simulink model "model_graphicSim"  (R2022a)
settings: Solver=FixedStepAuto  StartTime=0.0  StopTime=inf  RelTol=1e-3
values from neighbouring files (symbols this model uses):
  A = 9    [A_circuit_V2_25000.mat]    (also in A_circuit_V2_3167.mat; A_circuit_V3_30000.mat; A_circuit_V3_60000.mat; Configuration.m)
  d = 699840    [A_circuit_V2_25000.mat]    (also in A_circuit_V2_3167.mat; A_circuit_V3_30000.mat; A_circuit_V3_60000.mat; Configuration.m)
  egoID = 1    [A_circuit_V2_25000.mat]    (also in A_circuit_V2_3167.mat; A_circuit_V3_30000.mat; A_circuit_V3_60000.mat; Configuration.m)
  frontDistCG = 3.7    [A_circuit_V2_25000.mat]    (also in A_circuit_V2_3167.mat; A_circuit_V3_30000.mat; A_circuit_V3_60000.mat; Configuration.m)
  gridvx = [-5 -4.72222222222 -4.44444444444 -4.16666666667 -3.88888888889 -3.61111111111 -3.33333333333 -3.05555555556 -2.77777777778 -2.5 0 0.277777777778 ... (70 elements, 10x7)]    [A_circuit_V2_25000.mat]    (also in A_circuit_V2_3167.mat; A_circuit_V3_30000.mat; A_circuit_V3_60000.mat; circuit_10000_P2.mat)
  gridvy = [-70 -68.4444444444 -66.8888888889 -65.3333333333 -63.7777777778 -62.2222222222 -60.6666666667 -59.1111111111 -57.5555555556 -56 -50 -48.4444444444 ... (70 elements, 10x7)]    [A_circuit_V2_25000.mat]    (also in A_circuit_V2_3167.mat; A_circuit_V3_30000.mat; A_circuit_V3_60000.mat; circuit_10000_P2.mat)
  gridx = [-85 -84.6666666667 -84.3333333333 -84 -83.6666666667 -83.3333333333 -83 -82.6666666667 -82.3333333333 -82 -55 -54.6666666667 ... (70 elements, 10x7)]    [A_circuit_V2_25000.mat]    (also in A_circuit_V2_3167.mat; A_circuit_V3_30000.mat; A_circuit_V3_60000.mat; circuit_10000_P2.mat)
  gridy = [-70 -69.3333333333 -68.6666666667 -68 -67.3333333333 -66.6666666667 -66 -65.3333333333 -64.6666666667 -64 -50 -49.3333333333 ... (70 elements, 10x7)]    [A_circuit_V2_25000.mat]    (also in A_circuit_V2_3167.mat; A_circuit_V3_30000.mat; A_circuit_V3_60000.mat; circuit_10000_P2.mat)
  gridyaw = [-504 -489.6 -475.2 -460.8 -446.4 -432 -417.6 -403.2 -388.8 -374.4 -360 -345.6 ... (70 elements, 10x7)]    [A_circuit_V2_25000.mat]    (also in A_circuit_V2_3167.mat; A_circuit_V3_30000.mat; A_circuit_V3_60000.mat; circuit_10000_P2.mat)
  lb_angSt = -1080    [A_circuit_V2_25000.mat]    (also in A_circuit_V2_3167.mat; A_circuit_V3_30000.mat; A_circuit_V3_60000.mat; Configuration.m = -900)
  lbvx = 0    [A_circuit_V2_25000.mat]    (also in A_circuit_V2_3167.mat; A_circuit_V3_30000.mat; A_circuit_V3_60000.mat; Configuration.m = -2)
  lbvy = -50    [A_circuit_V2_25000.mat]    (also in A_circuit_V2_3167.mat; A_circuit_V3_30000.mat; A_circuit_V3_60000.mat; Configuration.m = -20)
  lbx = -55    [A_circuit_V2_25000.mat]    (also in A_circuit_V2_3167.mat; A_circuit_V3_30000.mat; A_circuit_V3_60000.mat; Configuration.m = 0)
  lby = -50    [A_circuit_V2_25000.mat]    (also in A_circuit_V2_3167.mat; A_circuit_V3_30000.mat; A_circuit_V3_60000.mat; Configuration.m = 2)
  lbyaw = -90    [Configuration.m]    (also in Configuration_circuit.m = -360; Configuration_circuit_V2.m = -360; Configuration_curve.m = -360; Configuration_curve_2.m = -360)
  leftDistCG = 0.9    [A_circuit_V2_25000.mat]    (also in A_circuit_V2_3167.mat; A_circuit_V3_30000.mat; A_circuit_V3_60000.mat; Configuration.m)
  M = 5    [A_circuit_V2_25000.mat]    (also in A_circuit_V2_3167.mat; A_circuit_V3_30000.mat; A_circuit_V3_60000.mat; Configuration.m)
  N = 10    [A_circuit_V2_25000.mat]    (also in A_circuit_V2_3167.mat; A_circuit_V3_30000.mat; A_circuit_V3_60000.mat; Configuration.m)
  passo_steerang = 45    [A_circuit_V2_25000.mat]    (also in A_circuit_V2_3167.mat; A_circuit_V3_30000.mat; A_circuit_V3_60000.mat; Configuration.m = 180)
  passo_v = 0.5    [A_circuit_V2_25000.mat]    (also in A_circuit_V2_3167.mat; A_circuit_V3_30000.mat; A_circuit_V3_60000.mat; Configuration.m)
  retroDistCG = 1    [A_circuit_V2_25000.mat]    (also in A_circuit_V2_3167.mat; A_circuit_V3_30000.mat; A_circuit_V3_60000.mat; Configuration.m)
  safetyDist = 0.5    [A_circuit_V2_25000.mat]    (also in A_circuit_V2_3167.mat; A_circuit_V3_30000.mat; A_circuit_V3_60000.mat; Configuration.m)
  Ts = 0.1    [A_circuit_V2_25000.mat]    (also in A_circuit_V2_3167.mat; A_circuit_V3_30000.mat; A_circuit_V3_60000.mat; Configuration.m)
  ub_angSt = 1080    [A_circuit_V2_25000.mat]    (also in A_circuit_V2_3167.mat; A_circuit_V3_30000.mat; A_circuit_V3_60000.mat; Configuration.m = 900)
  ubvx = 25    [A_circuit_V2_25000.mat]    (also in A_circuit_V2_3167.mat; A_circuit_V3_30000.mat; A_circuit_V3_60000.mat; Configuration.m = 2)
  ubvy = 50    [A_circuit_V2_25000.mat]    (also in A_circuit_V2_3167.mat; A_circuit_V3_30000.mat; A_circuit_V3_60000.mat; Configuration.m = 20)
  ubx = 95    [A_circuit_V2_25000.mat]    (also in A_circuit_V2_3167.mat; A_circuit_V3_30000.mat; A_circuit_V3_60000.mat; Configuration.m = 25)
  uby = 50    [A_circuit_V2_25000.mat]    (also in A_circuit_V2_3167.mat; A_circuit_V3_30000.mat; A_circuit_V3_60000.mat; Configuration.m = 10)
  ubyaw = 90    [Configuration.m]    (also in Configuration_circuit.m = 360; Configuration_circuit_V2.m = 360; Configuration_curve.m = 360; Configuration_curve_2.m = 360)
  w = [0 0 0 0 0 0 0 0 0 0 0 0 ... (699840 elements, 699840x1)]    [A_circuit_V2_25000.mat]    (also in A_circuit_V2_3167.mat; A_circuit_V3_30000.mat; A_circuit_V3_60000.mat; circuit_10000_P2.mat)
  x_0 = 2*rand+19    [Configuration.m]    (also in Configuration_circuit.m = -30; Configuration_circuit_V2.m = 0; Configuration_curve.m = 5; Configuration_curve_2.m = 5)
  y_0 = -(3.5*rand+2)    [Configuration.m]    (also in Configuration_circuit.m = -(-20 - rand*6); Configuration_circuit_V2.m = -(-29.5 - rand*7); Configuration_curve.m = -(1-2.1*rand); Configuration_curve_2.m = -(1-2.1*rand))
undefined symbols (not defined in the file or in its folder): deg, driving, rad, s
libraries: drivingscenarioandsensors x17, simulink_extras x2, sim3dlib x1, sim3dautolib x1, aerolibconvert2 x1, vehdynlibsteering x1, autolibshared x1
(part 6 of 6)

== matlab function model_graphicSim/next_a ==
  data: s input; a1 output; gridx parameter; gridy parameter; gridvx parameter; gridvy parameter; gridyaw parameter; M parameter; N parameter; A parameter; d parameter; eps parameter; w parameter; a2 output
function [a1,a2] = eps_greedy(s, gridx, gridy, gridvx, gridvy, gridyaw, M, N, A, d, eps, w)

%s(5) = -s(5);

if rand < eps   % azione random
    a = randi(A); % da 1 a 9 se uso indice
else
    q = zeros(A, 1);
    for a = 1:A  % valuto tutte le azioni che posso prendere
        q(a) = w'*get_features(s, a, gridx, gridy, gridvx, gridvy, gridyaw, M, N, A, d); % approsimazione della funz qualità
    end        % pesi per vett features
    a = find(q == max(q), 1, 'first'); % scelgo quella con funz qualità massima
end

[b1,b2] = ind2sub([3 3],a);

% [1 2 3] vanno mappati su -1,0, con (-2)

if(b1 == 1)
    a1 = 1;
elseif(b1 == 2)
    a1 = 2;
else
    a1 = 3;
end

if(b2 == 1)
    a2 = 1;
elseif(b2 == 2)
    a2 = 2;
else
    a2 = 3;
end

end


function x = get_features(s, a, gridx, gridy, gridvx, gridvy, gridyaw, M, N, A, d)

%coder.extrinsic('assignin')

% numero celle, +1 perchè ne ho aggiunta una
%nCells = (M + 1)^4; % dimensione features per una cella
%d = A*N*nCells; % dimensione vettore pesi da aggiornare
x = zeros(d, 1);
% va modificaro sta dimension var
for ii = 1 : N
    xxx = gridx(ii, :);
    yyy = gridy(ii, :);
    vxvxvx = gridvx(ii, :);
    vyvyvy = gridvy(ii, :);
    yawyawyaw = gridyaw(ii, :);
    % capire in quale cella mi trovo, trovo indice lungo x e lungo y
    ix = find(s(1) >= xxx(1:end-1) & s(1) <= xxx(2:end), 1, 'first');
    iy = find(s(2) >= yyy(1:end-1) & s(2) <= yyy(2:end), 1, 'first');
    ivx = find(s(3) >= vxvxvx(1:end-1) & s(3) <= vxvxvx(2:end), 1, 'first');
    ivy = find(s(4) >= vyvyvy(1:end-1) & s(4) <= vyvyvy(2:end), 1, 'first');
    iyaw = find(s(5) >= yawyawyaw(1:end-1) & s(5) <= yawyawyaw(2:end), 1, 'first');

    % a_ind = sub2ind([3 3],a(1),a(2)); non serve gli passo indice poi da
    % indice a azione quando la uso in dinamica
    % dato doppia dim dell'azione devo subind anche a ???

    % debug
    %pippo = struct('ix',{ix},'iy', {iy},'ivx', {ivx},'ivy', {ivy},'ii', {ii},'a', {a},'s', {s});
    %assignin("base","pippo",pippo);
    % ind = sub2ind([M + 1, M + 1, M + 1, M + 1, N, A], ix, iy, ivx, ivy, ii, a);
    ind = sub2ind([M + 1, M + 1, M + 1, M + 1, M + 1, N, A], ix, iy, ivx, ivy, iyaw, ii, a);

    x(ind) = 1; % valore corrispondente alla cella
    % vett features ha un 1 per ogni griglia
end
end

== matlab function model_graphicSim/Reward ==
  data: sp output; next_state input; RadR input; RadF input; RadSx input; RadDx input; camL_L input; camF_L input; camR_L input; r output; isTerminal output; safetyDist parameter; leftDistCG parameter; frontDistCG parameter; retroDistCG parameter; ubx parameter; lbx parameter; uby parameter; ubyaw parameter; lbyaw parameter; lby parameter
% sensori camera hanno difficoltà con ostacoli ravvicinati -> provare radar
function [sp , r, isTerminal] = reward(next_state, RadR, RadF, RadSx, RadDx, camL_L, camF_L, camR_L, safetyDist, leftDistCG, frontDistCG, retroDistCG, ubx, lbx, uby, ubyaw, lbyaw, lby)

% isTerminal quadno crash, quando fuori da ambiente -> r = r - 1000
% isTerminal qunado raggiungo distanza limite dal bordo -> r = 0
% altrimenti r = r - 1

% CG centro asse posteriore

sp = next_state;

% controllo posizione non fuori dai limiti (next_state = [x y vx vy])
% limiti ambiente statici, definirli come parametri da workspace
% if((next_state(1) < 0) || (next_state(1) > 25) || (next_state(2) < -10) || (next_state(2) > 10))
%     
%     %fatti cosi sto considerando il centro ma la mia macchina ha delle dimensioni e anche orientamento yaw
%     % se considero misure CG alla fine sto considerando spazio più grande
%     % 
%     r = -1000;
%     isTerminal = 1;
%     return
% end

%fatti cosi sto considerando il centro ma la mia macchina ha delle dimensioni e anche orientamento yaw
% se considero misure CG alla fine sto considerando spazio più grande
if((next_state(1) < lbx) )% || (next_state(1) > 25) || (next_state(2) < -10) || (next_state(2) > 10))
    sp(1) = lbx;
    r = -1000;
    isTerminal = 1;
    return
elseif(next_state(1) > ubx)
    sp(1) = ubx;
    r = -1000;                 % questi numeri vanno sostituiti con i parametri da workspace
    isTerminal = 1;
    return
elseif(next_state(2) < lby)
    sp(2) = lby;
    r = -1000;
    isTerminal = 1;
    return
elseif(next_state(2) > uby)
    sp(2) = uby;
    r = -1000;
    isTerminal = 1;
    return
end
% controllo su yaw
if(next_state(5) > ubyaw )
    sp(5) = ubyaw;
    r = -1000;
    isTerminal = 1;
    return
elseif(next_state(5) < lbyaw )
    sp(5) = lbyaw;
    r = -1000;
    isTerminal = 1;
    return
end


%%%%%%%%%%%%%%%%%%%%%%%%%%%%%%%%%%%%%%%%%%%%%%%%%%%%%%%%%%%%%%%%%%%%%%%%%%%
% Per misure sensori verificare distanza da CG
% Sistema di riferimento centrato e fissato nel CG del veicolo
% front e retro(neg) lungo x, lateral lungo y -> misure da considerare
% abs sulle misure
%%%%%%%%%%%%%%%%%%%%%%%%%%%%%%%%%%%%%%%%%%%%%%%%%%%%%%%%%%%%%%%%%%%%%%%%%%%
% per ogni cam ho una serie di detection

% CONTROLLO CRASH  questo lo faccio per ultimo
% utilizzo abs sulle misure mi interessa val assoluto
% Object detection sensore non rileva oggetto non mi ritorna cella, control
% dimensioni veicolo diatnze da CG

% FRONT CRASH
%camF.Detections(i).Measurement(1) % x 
%camF.Detections(i).Measurement(2) % y
i = 1;
while(RadF.Detections(i).Measurement(1) ~= 0) % posizione ritornata va triangolata ???
    % Front controllo su x
    if((abs(RadF.Detections(i).Measurement(1)) - frontDistCG) < safetyDist)
        r = -1000;
        isTerminal = 1;
        return
    end
    i = i + 1;
end 
%for i=1:size(camF.Detections(i))
% RETRO CRASH
i = 1;
while(RadR.Detections(i).Measurement(1) ~= 0) % posizione ritornata va triangolata ???
    % Front controllo su x
    if((abs(RadR.Detections(i).Measurement(1)) - retroDistCG) < safetyDist)
        r = -1000;
        isTerminal = 1;
        return
    end
    i = i + 1;
end 

%LEFT CRASH
i = 1;
while(RadSx.Detections(i).Measurement(2) ~= 0) % posizione ritornata va triangolata ???
    % Front controllo su x
    if((abs(RadSx.Detections(i).Measurement(2)) - leftDistCG) < safetyDist)
        r = -1000;
        isTerminal = 1;
        return
    end
    i = i + 1;
end

%RIGHT CRASH
i = 1;
while(RadDx.Detections(i).Measurement(2) ~= 0) % posizione ritornata va triangolata ???
    % Front controllo su x
    if((abs(RadDx.Detections(i).Measurement(2)) - leftDistCG) < safetyDist)
        r = -1000;
        isTerminal = 1;
        return
    end
    i = i + 1;
end

% Controllo sulle 3 cam la lane dist
% aznche qui devo togliere distanza fissa CG dalla cam che rileva
lateral_offset = camL_L.LaneBoundaries(1).LateralOffset;

if(isnan(lateral_offset))
    lateral_offset = camR_L.LaneBoundaries(1).LateralOffset;
    if(isnan(lateral_offset))
        lateral_offset = camF_L.LaneBoundaries(1).LateralOffset;
        if(isnan(lateral_offset))
%%%%%%%%%%%%%%%%%%%%%%%%%%%%%%%%%%%%%%%%%%%%%%%%%%%%%%%%%%%%%%%%%%%%%%%%%%            
            lateral_offset = 5; % utilizzo lect precedente                  % SISTEMARE QUI PROB Nan 
%%%%%%%%%%%%%%%%%%%%%%%%%%%%%%%%%%%%%%%%%%%%%%%%%%%%%%%%%%%%%%%%%%%%%%%%%%            
        end
    end
end

% CONTROLLO STATO TERMINALE arrivo a dist min dal bordo
% successivame controllo se vado oltre la linea
%if( (abs(lateral_offset) - leftDistCG) < safetyDist + 0.2 )

yaw_calc = abs(sp(5));
if( ((abs(lateral_offset) - leftDistCG) <= 1) && (yaw_calc <= 30))   % modifiche qui
    r = 0;
    isTerminal = 1;
    return
end

% if((abs(lateral_offset) - leftDistCG) < 1)                % modifiche qui
%     r = -1000;
%     isTerminal = 1;
%     return
% end

% problema se auto gira e legge linea dall'altra parte controllo yaw vlong
% controllo diff posizioni e vedo in che direzione si muove


%Proviamo singola camera laterale con misura da CG
% successivamente proveremo due camere posizionate sulle ruote

r = -1 - abs(lateral_offset);
isTerminal = 0;

== matlab function model_graphicSim/MATLAB Function ==
  data: u input; y output
function y = fcn(u)

y = u.Detections(1).Measurement(1);

== matlab function model_graphicSim/Vehicle/MATLAB Function ==
  data: yaw input; yaw_limit output
function yaw_limit = fcn(yaw)

if(yaw > 360)
    yaw_limit = yaw - 360;

elseif(yaw < -360)
     yaw_limit = yaw + 360;
else
    yaw_limit = yaw;
end

end

== matlab function model_graphicSim/Scenario Simulation/Pack Ego Actor ==
  data: pos input; a output Bus: BusActors1Actors size=1; vel input; yaw input; yawRate input; egoID input
function a = packEgo(pos,vel,yaw,yawRate,egoID)
% Pack ego information into a single ego actor bus
%
% Imoprtant note:
% Output is a bus of type BusActorsActors. This is the same bus used by the
% Scenario Reader to output an individual actor. If you change the
% output bus name of Scenario Reader change the output bus name here
% as well by clicking on 'Edit Data' in the menu above.

a = struct(...
    'ActorID',egoID,...
    'Position', [pos(1) pos(2) 0], ...
    'Velocity', [vel(1) vel(2) 0], ...
    'Roll', 0, ...
    'Pitch', 0, ...
    'Yaw', yaw, ...
    'AngularVelocity', [0 0 yawRate]);

== matlab function model_graphicSim/debug_objDet ==
  data: u input; y output; o input; y1 output; y2 output; y3 output
function [y, y1,y2,y3] = fcn(u,o)

%y = u.LaneBoundaries(1).LateralOffset;
%y = size(o.Detections(1).Measurement);

%y = u.LaneBoundaries(1).LateralOffset;
%y1 = u.LaneBoundaries(2).LateralOffset;
%y2 = u.LaneBoundaries(3).LateralOffset;
%y3 = u.LaneBoundaries(4).LateralOffset;
%if(o.Detections(1).Measurement == zeros(1,6))
%    y = 555;
%end
 y = size(o.Detections);
 y1 = o.Detections(1).Measurement;
 y2 = o.Detections(2).Measurement;
 y3 = o.Detections(13).Measurement;


% detection nmero elementi rilevati
% controllo tutti quelli diversi da 6 zeri , no detection tutte zero
%y1= 1;
